simulink model "P1Simulink"  (R2023b)
settings: Solver=VariableStepAuto  StartTime=0.0  StopTime=25  FixedStep=1  RelTol=1e-3
undefined symbols (not defined in the file): DiscIntNeverNeededParam, K, kw, R, tau, Ts, wd
settings Model: Creator=rpl  LastModifiedBy=rpl

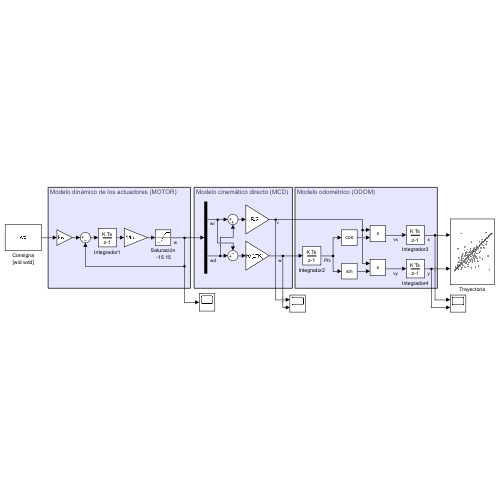
[thumbnail: Simulink's stored preview of the top-level diagram]
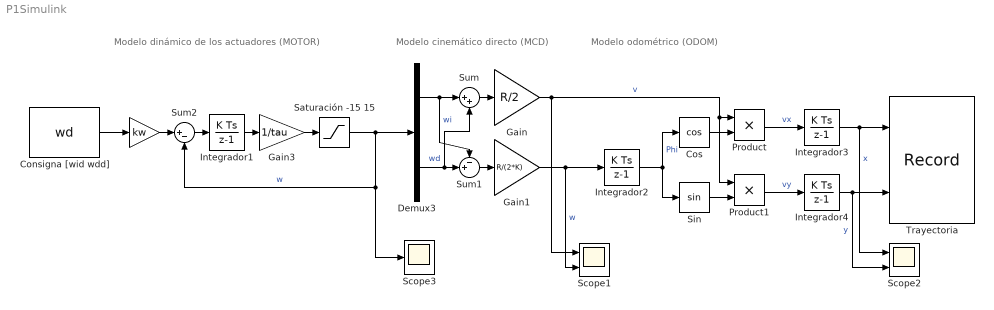
== system P1Simulink ==
  note: Modelo odométrico (ODOM)
  note: Modelo cinemático directo (MCD)
  note: Modelo dinámico de los actuadores (MOTOR)
  " " : Gain  Gain=kw
  Consigna [wid wdd] : Constant  Value=wd  SampleTime=Ts
  Cos : Trigonometry  Operator=cos
  Demux3 : Demux  Outputs=2
  Gain : Gain  Gain=R/2
  Gain1 : Gain  Gain=R/(2*K)
  Gain3 : Gain  Gain=1/tau
  Integrador{1..4} (4 alike) : DiscreteIntegrator  SampleTime=-1  ICPrevOutput=DiscIntNeverNeededParam  ICPrevScaledInput=DiscIntNeverNeededParam
  Product : Product
  Product1 : Product
  Saturación -15 15 : Saturate  UpperLimit=15  LowerLimit=-15
  Scope1 : Scope  NumInputPorts=2
  Scope2 : Scope  NumInputPorts=2
  Scope3 : Scope
  Sin : Trigonometry
  Sum : Sum  Inputs=|++
  Sum1 : Sum  Inputs=-+|
  Sum2 : Sum  Inputs=|+-
  Trayectoria : Record  FileSettingsInternal="{\"entries\":[{\"content\":{\"excelSettings\":{\"content\":{},\"type\":\"Streamout.ExcelSettings\"}},\"type\":\"Streamout.FileSettingStorage\",\"uuid\":\"\"}],\"packageUris\":[\"http:\\/\\/schema.mathworks.com\\/mf0\\/streamout_blocks\\/R2020a\"],\"version\":\"1.0\"}"  Layout=[1 1]  SignalsInternal="{\"entries\":[{\"content\":{\"signals\":[{\"content\":{\"blockPath\":[],\"dimensions\":[1],\"domain\":\"\",\"lineColor\":\"#fe330a\",\"plots\":[ 1 ],\"port\":1,\"sid\":[\"\"],\"signalID\":1,\"signalName\":\"x\"},\"type\":\"RecordBlkView.Signal\",\"uuid\":\"\"},{\"content\":{\"blockPath\":[],\"dimensions\":[1],\"domain\":\"\",\"lineColor\":\"#22b573\",\"plots\":[ 1 ],\"port\":2,\"sid\":[\"\"],\"signalID\":2,\"signalName\":\"y\"},\"type\":\"RecordBlkView.Signal\",\"uuid\":\"\"}]},\"type\":\"RecordBlkView.InputSignals\",\"uuid\":\"\"}],\"packageUris\":[\"http:\\/\\/schema.mathworks.com\\/mf0\\/streamout_blocks\\/R2020a\"],\"version\":\"1.0\"}"  VisualizationBindings="{\"xyplotplugin\":{\"info\":[{\"series\":[{\"bindingParametersList\":[{\"parameter\":\"X-Axis\",\"signalID\":1,\"signalName\":\"x\"},{\"parameter\":\"Y-Axis\",\"signalID\":2,\"signalName\":\"y\"}],\"seriesID\":0}],\"subplotID\":1}]}}"  CompatibilityTag=XY
  wires:
  Sum/1 -> Gain/1
  Sum1/1 -> Gain1/1
  Integrador2/1 -> Cos/1, Sin/1  "Phi"
  Cos/1 -> Product/2
  Sin/1 -> Product1/2
  Product/1 -> Integrador3/1  "vx"
  Product1/1 -> Integrador4/1  "vy"
  Integrador3/1 -> Scope2/1, Trayectoria/1  "x"
  Integrador4/1 -> Scope2/2, Trayectoria/2  "y"
  Gain/1 -> Product1/1, Product/1, Scope1/1  "v"
  Gain1/1 -> Integrador2/1, Scope1/2  "w"
  Consigna [wid wdd]/1 -> " "/1
  " "/1 -> Sum2/1
  Sum2/1 -> Integrador1/1
  Gain3/1 -> Saturación -15 15/1
  Saturación -15 15/1 -> Demux3/1, Scope3/1, Sum2/2  "w"
  Integrador1/1 -> Gain3/1
  Demux3/1 -> Sum1/1, Sum/1  "wi"
  Demux3/2 -> Sum/2, Sum1/2  "wd"
